simulink model "EvitaParedes"  (R2023b)
settings: Solver=FixedStepDiscrete  StartTime=0.0  StopTime=Inf  FixedStep=0.01  RelTol=1e-3  EnableMultiTasking=on
settings Model: ExtModeTrigDuration=2  Creator=Andrés  LastModifiedBy=Andrés
settings OptimizationCC: EnhancedBackFolding=on  PassReuseOutputArgsAs=Individual arguments  ZeroExternalMemoryAtStartup=off  ZeroInternalMemoryAtStartup=off  MaxStackSize=64  OptimizeBlockOrder=speed  DifferentSizesBufferReuse=on  OptimizationCustomize=off  EfficientTunableParamExpr=on
settings DebuggingCC: ParameterOverflowMsg=none  ParameterTunabilityLossMsg=error
settings HardwareCC: ProdBitPerInt=16  ProdBitPerPointer=16  ProdBitPerSizeT=16  ProdBitPerPtrDiffT=16  ProdLargestAtomicFloat=None  ProdWordSize=8  ProdHWDeviceType=Atmel->AVR  UseEmbeddedCoderFeatures=off  UseSimulinkCoderFeatures=off
settings SFSimCC: MATLABDynamicMemAlloc=off
settings RTWCC: Description=Embedded Coder  SystemTargetFile=ert.tlc  HardwareBoard=Arduino Mega 2560  TemplateMakefile=ert_default_tmf  Toolchain=Arduino AVR  BuildConfiguration=Faster Runs
settings CodeAppCC: ForceParamTrailComments=on  IgnoreCustomStorageClasses=off  OperatorAnnotations=on  SimulinkDataObjDesc=on  SFDataObjDesc=on  MangleLength=10  InsertBlockDesc=on
settings ERTTargetCC: SupportContinuousTime=on  SupportNonInlinedSFcns=on  SupportVariableSizeSignals=on  ExtModeTransport=3  ExtModeStaticAlloc=on  ExtModeAutomaticAllocSize=off  ExtModeStaticAllocSize=2048  ExtModeMexFile=ext_xcp  ExtModeIntrfLevel=Level2 - Open

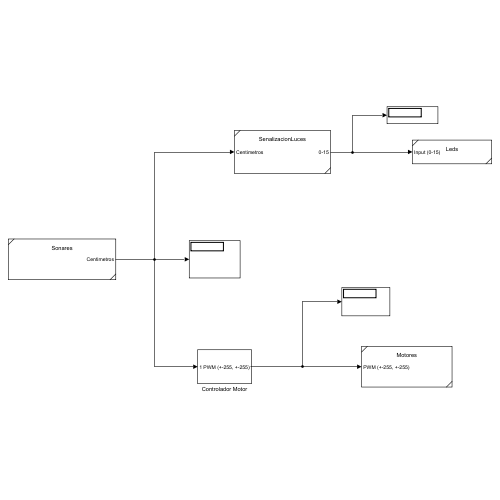
[thumbnail: Simulink's stored preview of the top-level diagram]
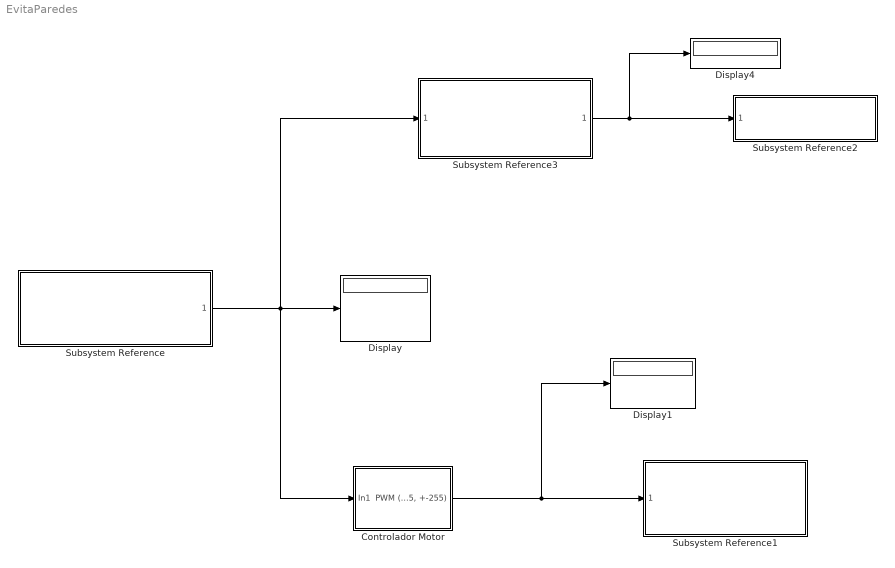
== system EvitaParedes ==
  Controlador Motor : Subsystem
  Display : Display
  Display1 : Display
  Display4 : Display
  Subsystem Reference : Subsystem  ReferencedSubsystem=Sonares
  Subsystem Reference1 : Subsystem  ReferencedSubsystem=Motores
  Subsystem Reference2 : Subsystem  ReferencedSubsystem=Leds
  Subsystem Reference3 : Subsystem  ReferencedSubsystem=SenalizacionLuces
  wires:
  Controlador Motor/1("PWM (+-255, +-255)") -> Subsystem Reference1/1, Display1/1
  Subsystem Reference3/1 -> Display4/1, Subsystem Reference2/1
  Subsystem Reference/1 -> Subsystem Reference3/1, Controlador Motor/1(In1), Display/1

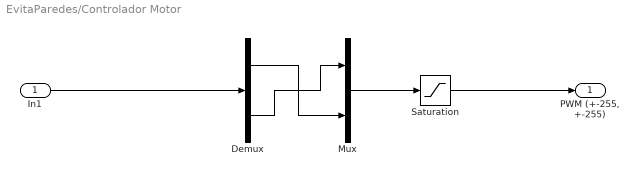
== system EvitaParedes/Controlador Motor ==
  In1 : Inport
  Demux : Demux  Outputs=2
  Mux : Mux  Inputs=2
  Saturation : Saturate  UpperLimit=180  LowerLimit=-180
  "PWM (+-255, +-255)" : Outport
  wires:
  Demux/1 -> Mux/2
  Demux/2 -> Mux/1
  In1/1 -> Demux/1
  Mux/1 -> Saturation/1
  Saturation/1 -> "PWM (+-255, +-255)"/1
